simulink model "system_model"  (R2022b)
settings: Solver=ode4  StartTime=0.0  StopTime=3000*10  FixedStep=2  RelTol=1e-3
settings Model: Creator=hurtado  LastModifiedBy=hurta
settings DebuggingCC: UnconnectedInputMsg=warning  UnconnectedOutputMsg=warning  UnconnectedLineMsg=warning
settings ModelReferenceCC: EnableRefExpFcnMdlSchedulingChecks=on
settings RTWCC: DLArmComputeVersion=19.05

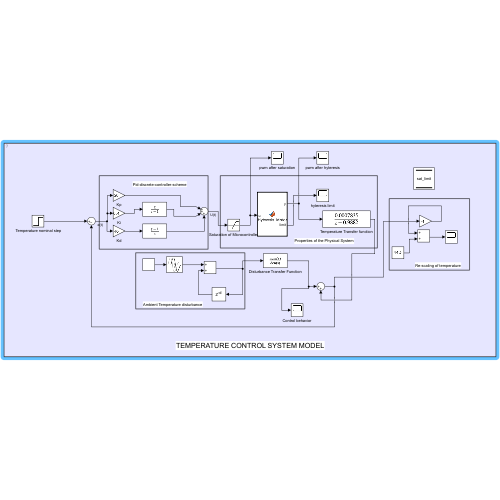
[thumbnail: Simulink's stored preview of the top-level diagram]
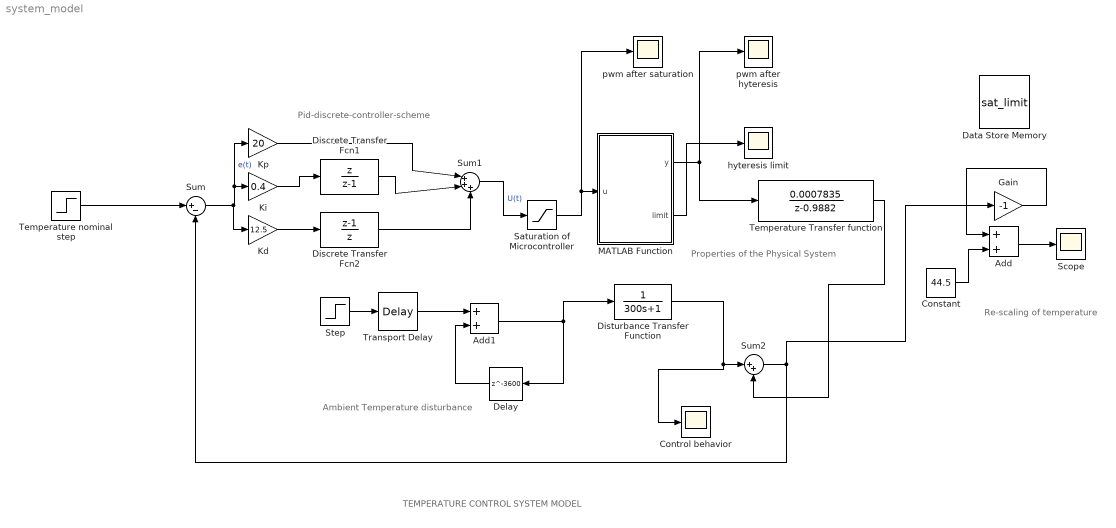
== system system_model ==
  note: TEMPERATURE CONTROL SYSTEM MODEL
  note: Properties of the Physical System
  note: Pid-discrete-controller-scheme
  note: Re-scaling of temperature
  note: Ambient Temperature disturbance
  " Temperature nominal step" : Step  Time=0  After=3.5  SampleTime=2
  Add : Sum
  Add1 : Sum
  Constant : Constant  Value=44.5
  Control behavior : Scope
  Data Store Memory : DataStoreMemory  DataStoreName=sat_limit  ReadBeforeWriteMsg=warning  WriteAfterWriteMsg=warning  WriteAfterReadMsg=warning  InitialValue=160  ShowAdditionalParam=off  OutDataTypeStr=double
  Delay : Delay  DelayLength=3600  InitialCondition=0
  Discrete Transfer Fcn1 : DiscreteTransferFcn  Numerator=[1 0]  Denominator=[1 -1]
  Discrete Transfer Fcn2 : DiscreteTransferFcn  Numerator=[1 -1]  Denominator=[1 0]
  Disturbance Transfer Function : TransferFcn  Denominator=[300 1]
  Gain : Gain  Gain=-1
  Kd : Gain  Gain=12.5
  Ki : Gain  Gain=0.4
  Kp : Gain  Gain=20
  MATLAB Function : MATLAB Function  TreatAsAtomicUnit=on
  Saturation of Microcontroller : Saturate  UpperLimit=255  LowerLimit=0
  Scope : Scope
  Step : Step  Time=100  After=-1.0  SampleTime=0
  Sum : Sum  Inputs=|+-
  Sum1 : Sum  Inputs=|+++
  Sum2 : Sum  Inputs=|++
  Temperature Transfer function : DiscreteTransferFcn  Numerator=[0.0007835]  Denominator=[1 -0.9882]
  Transport Delay : TransportDelay  DelayTime=3600
  hyteresis limit : Scope
  pwm after hyteresis : Scope
  pwm after saturation : Scope
  wires:
  Temperature Transfer function/1 -> Sum2/2
  Kp/1 -> Sum1/1
  Ki/1 -> Discrete Transfer Fcn1/1
  Kd/1 -> Discrete Transfer Fcn2/1
  Discrete Transfer Fcn1/1 -> Sum1/2
  Discrete Transfer Fcn2/1 -> Sum1/3
  " Temperature nominal step"/1 -> Sum/1
  Constant/1 -> Add/2
  Gain/1 -> Add/1
  Sum/1 -> Kd/1, Ki/1, Kp/1  "e(t)"
  MATLAB Function/1(y) -> pwm after hyteresis/1, Temperature Transfer function/1
  Saturation of Microcontroller/1 -> MATLAB Function/1(u), pwm after saturation/1
  MATLAB Function/2(limit) -> hyteresis limit/1
  Sum2/1 -> Gain/1, Sum/2
  Add1/1 -> Delay/1, Disturbance Transfer Function/1
  Delay/1 -> Add1/2
  Step/1 -> Transport Delay/1
  Transport Delay/1 -> Add1/1
  Add/1 -> Scope/1
  Sum1/1 -> Saturation of Microcontroller/1  "U(t)"
  Disturbance Transfer Function/1 -> Control behavior/1, Sum2/1

== matlab function system_model/MATLAB Function ==
  settings: updateMethod=DISCRETE
  data: u input; y output; sat_limit data_store_memory; limit output
function [y,limit]  = Hyteresis_Motor(u)
global sat_limit;
if u>160
    sat_limit = 70;
elseif u<70
    sat_limit = 300;
end
if (u>sat_limit)
    u=u;
else
    u=0;
end
y = u;
limit = sat_limit;
